simulink model "maglev_linearizado"  (R2025b)
settings: Solver=VariableStepAuto  StartTime=0.0  StopTime=10.0  RelTol=1e-3
undefined symbols (not defined in the file): Kd, Ki, Kp, u0
settings Model: Creator=gusta  LastModifiedBy=gusta

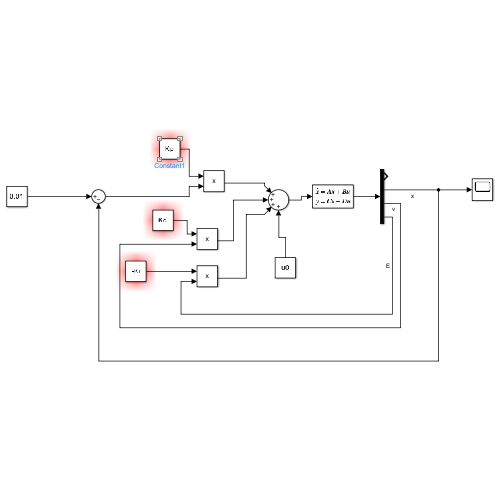
[thumbnail: Simulink's stored preview of the top-level diagram]
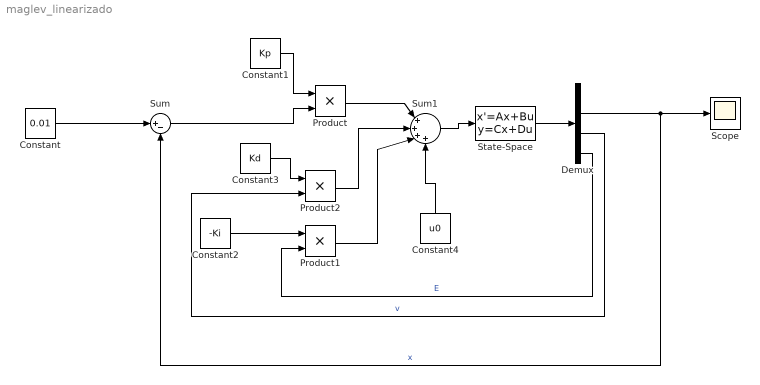
== system maglev_linearizado ==
  Constant : Constant  Value=0.01
  Constant1 : Constant  Value=Kp
  Constant2 : Constant  Value=-Ki
  Constant3 : Constant  Value=Kd
  Constant4 : Constant  Value=u0
  Demux : Demux
  Product : Product
  Product1 : Product
  Product2 : Product
  Scope : Scope
  State-Space : StateSpace  InitialCondition=0
  Sum : Sum  Inputs=|+-
  Sum1 : Sum  Inputs=|++++
  wires:
  Constant/1 -> Sum/1
  State-Space/1 -> Demux/1
  Demux/2 -> Scope/1, Sum/2  "x"
  Constant1/1 -> Product/1
  Sum/1 -> Product/2
  Sum1/1 -> State-Space/1
  Product/1 -> Sum1/1
  Constant2/1 -> Product1/1
  Constant3/1 -> Product2/1
  Demux/3 -> Product2/2  "v"
  Demux/4 -> Product1/2  "E"
  Product2/1 -> Sum1/2
  Product1/1 -> Sum1/3
  Constant4/1 -> Sum1/4
